simulink model "Lab6dff"  (R2016b)
settings: Solver=FixedStepAuto  StartTime=0.0  StopTime=20  FixedStep=0.01  RelTol=1e-3  EnableMultiTasking=on
values from neighbouring files (symbols this model uses):
  A = [0 a12 0 0;0 a22 a23 0;0 0 0 a34;0 a42 a43 0]    [Lab6d.m]    (also in data.mat = [0 0 0 0 1 -6.81227956989 0 15.4730759462 0 -1.49574193548 0; data2.mat = [0 0 0 0 1 -6.81227956989 0 15.4730759462 0 -1.49574193548 0; data3.mat = [0 0 0 0 1 -6.81227956989 0 15.4730759462 0 -1.49574193548 0; data4.mat = [0 0 0 0 1 -6.81227956989 0 15.4730759462 0 -1.49574193548 0)
  ang_thresh = 10*pi/180    (= 0.174532925199)    [Lab6d.m]    (also in data.mat; data2.mat; data3.mat; data4.mat)
  B = [0;b2;0;b4]    [Lab6d.m]    (also in data.mat = [0 1.52258064516 0 -3.45831460894]; data2.mat = [0 1.52258064516 0 -3.45831460894]; data3.mat = [0 1.52258064516 0 -3.45831460894]; data4.mat = [0 1.52258064516 0 -3.45831460894])
  C = [1 0 0 0;0 0 1 0]    [Lab6d.m]    (also in data.mat = [1  0  0  0; 0  0  1  0]; data2.mat = [1  0  0  0; 0  0  1  0]; data3.mat = [1  0  0  0; 0  0  1  0]; data4.mat = [1  0  0  0; 0  0  1  0])
  c_lp = 0.016    [Lab6d.m]    (also in data.mat; data2.mat; data3.mat; data4.mat)
  K = lqr(A,B,Q,R)    [Lab6d.m]    (also in data.mat = [-20 -39.3881221212 -301.165512499 -28.5227586286]; data2.mat = [-20 -39.3881221212 -301.165512499 -28.5227586286]; data3.mat = [-20 -39.3881221212 -301.165512499 -28.5227586286]; data4.mat = [-20 -39.3881221212 -301.165512499 -28.5227586286])
  K_pump = 300    [Lab6d.m]    (also in data.mat; data2.mat; data3.mat; data4.mat)
  L = place(A',C',po)'    [Lab6d.m]    (also in data.mat = [16.1595183214  -2.37669395577; 254.97799534  -5.48182894616; data2.mat = [16.1595183214  -2.37669395577; 254.97799534  -5.48182894616; data3.mat = [16.1595183214  -2.37669395577; 254.97799534  -5.48182894616; data4.mat = [16.1595183214  -2.37669395577; 254.97799534  -5.48182894616)
  ref = [0; 0; 0; 0]    [Lab6d.m]    (also in data.mat = [0 0 0 0]; data2.mat = [0 0 0 0]; data3.mat = [0.3 0 0 0]; data4.mat = [0.3 0 0 0])
  SAT = 4    [Lab6d.m]    (also in data.mat; data2.mat; data3.mat; data4.mat)
undefined symbols (not defined in the file or in its folder): HIL
libraries: quarc_library x3
settings Model: SimulationMode=external  Creator=ee128-aac  LastModifiedBy=ee105-abq
settings SolverCC: PositivePriorityOrder=on
settings RTWCC: SystemTargetFile=quarc_win64.tlc  TemplateMakefile=quarc_default_tmf  Description=QUARC Win64 Target
settings STFCustomTargetCC: TargetPreCompLibLocation=C:\PROGRA~3\QUARC\lib\2016b\win64\release  TargetLangStandard=C99 (ISO)  ConcurrentExecutionCompliant=on  SystemTargetFile=quarc_win64.tlc
settings GRTTargetCC: TargetPreCompLibLocation=C:\PROGRA~3\QUARC\lib\2016b\win64\release  ParMdlRefBuildCompliant=off  CompOptLevelCompliant=off  CombineOutputUpdateFcns=off  MatFileLogging=off  CPPClassGenCompliant=off  GRTInterface=on  UseToolchainInfoCompliant=off  ExtMode=on  ExtModeMexFile=quarc_comm

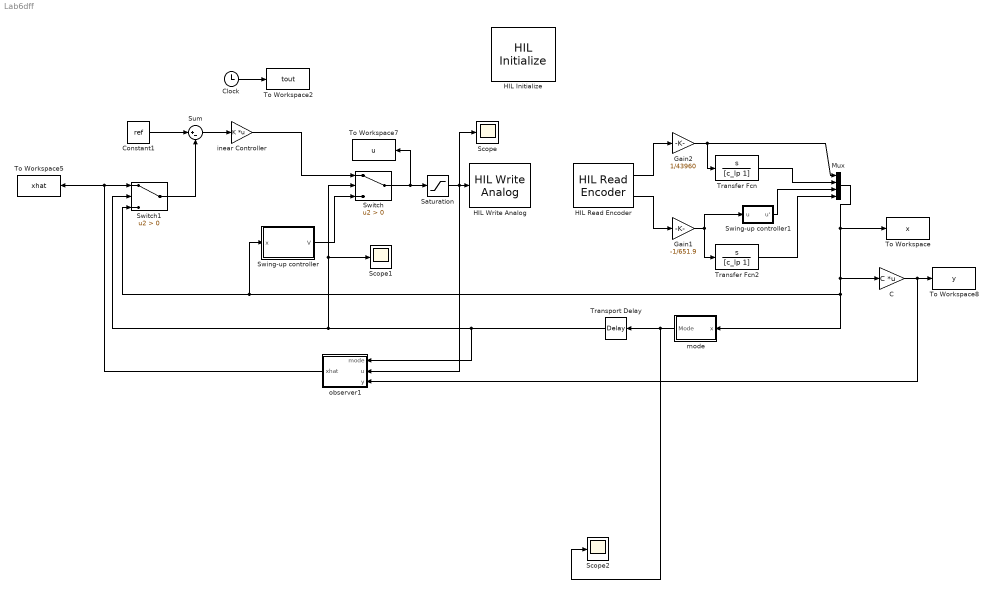
== system Lab6dff ==
  "C " : Gain  Gain=C  Multiplication=Matrix(K*u)
  Clock : Clock
  Constant1 : Constant  Value=ref
  Gain1 : Gain  Gain=-1/651.9
  Gain2 : Gain  Gain=1/43960
  HIL Initialize : quarc_library/Data Acquisition/Generic/Configuration/HIL Initialize  object_name=HIL-1  board_type=q4  board_number=0  board_options=""  exclusive=off  active=on  hardware_clocks=[0:1]  clock_modes=[0 0]  initial_clock_frequencies=[]  set_clock_params_at_start=on  set_clock_params_at_switch_in=off  set_clock_frequencies_at_start=off  set_clock_frequencies_at_switch_in=off  analog_input_channels=[0:3]  analog_input_configurations=[]  analog_input_maximums=10  analog_input_minimums=-10  set_analog_input_params_at_start=off  set_analog_input_params_at_switch_in=off  analog_output_channels=[0:3]  analog_output_maximums=[10]  analog_output_minimums=[-10]  initial_analog_outputs=[0]  final_analog_outputs=[0]  watchdog_analog_outputs=0  set_analog_output_params_at_start=on  set_analog_output_params_at_switch_in=off  set_analog_outputs_at_start=on  set_analog_outputs_at_switch_in=off  set_analog_outputs_at_terminate=on  set_analog_outputs_at_switch_out=off  set_analog_outputs_on_watchdog=off  digital_input_channels=[]  digital_output_channels=[]  digital_output_configuration=[]  initial_digital_outputs=[1]  final_digital_outputs=[1]  watchdog_digital_outputs=[2]  set_digital_output_params_at_start=off  set_digital_output_params_at_switch_in=off  set_digital_outputs_at_start=on  set_digital_outputs_at_switch_in=off  set_digital_outputs_at_terminate=on  set_digital_outputs_at_switch_out=off  set_digital_outputs_on_watchdog=off  encoder_channels=[0:3]  quadrature=[4]  encoder_filter_frequency=(1/60e-9)/1  initial_encoder_counts=[0]  set_encoder_params_at_start=on  set_encoder_params_at_switch_in=off  set_encoder_counts_at_start=on  set_encoder_counts_at_switch_in=off  pwm_channels=[]  pwm_modes=[0]  pwm_frequency=(1/60e-9)/1024  pwm_configuration=[]  pwm_alignment=[]  pwm_polarity=[]  pwm_leading_deadband=[]  pwm_trailing_deadband=[]  initial_pwm_outputs=[0]  final_pwm_outputs=[0]  watchdog_pwm_outputs=[]  set_pwm_params_at_start=on  set_pwm_params_at_switch_in=off  set_pwm_outputs_at_start=on  set_pwm_outputs_at_switch_in=off  set_pwm_outputs_at_terminate=on  set_pwm_outputs_at_switch_out=off  set_pwm_outputs_on_watchdog=off  other_output_channels=[]  initial_other_outputs=[]  final_other_outputs=[]  watchdog_other_outputs=[]  set_other_outputs_at_start=off  set_other_outputs_at_switch_in=off  set_other_outputs_at_terminate=off  set_other_outputs_at_switch_out=off  set_other_outputs_on_watchdog=off
  HIL Read Encoder : quarc_library/Data Acquisition/Generic/Immediate I//O/HIL Read Encoder  object_name=HIL-1  channels=[0:1]  sample_time=qc_get_step_size  active=on  vector_output=off  data_type_mode=Inherit via back propagation  data_type=double
  HIL Write Analog : quarc_library/Data Acquisition/Generic/Immediate I//O/HIL Write Analog  object_name=HIL-1  channels=[0]  sample_time=-1  active=off  vector_input=off
  Mux : Mux
  Saturation : Saturate  UpperLimit=6  LowerLimit=-6
  Scope : Scope
  Scope1 : Scope
  Scope2 : Scope
  Sum : Sum  Inputs=|+-
  Swing-up controller : Subsystem
  Swing-up controller1 : Subsystem
  Switch : Switch  Criteria=u2 > Threshold
  Switch1 : Switch  Criteria=u2 > Threshold
  To Workspace : ToWorkspace  VariableName=x  SampleTime=-1
  To Workspace2 : ToWorkspace  VariableName=tout  SampleTime=-1
  To Workspace5 : ToWorkspace  VariableName=xhat  SampleTime=-1
  To Workspace7 : ToWorkspace  VariableName=u  SampleTime=-1
  To Workspace8 : ToWorkspace  VariableName=y  SampleTime=-1
  Transfer Fcn : TransferFcn  Numerator=[1 0]  Denominator=[c_lp 1]
  Transfer Fcn2 : TransferFcn  Numerator=[1 0]  Denominator=[c_lp 1]
  Transport Delay : TransportDelay  DelayTime=0.25
  "inear Controller " : Gain  Gain=K  Multiplication=Matrix(K*u)
  mode : Subsystem
  observer1 : Subsystem
  wires:
  Saturation/1 -> observer1/2(u), HIL Write Analog/1, Scope/1
  HIL Read Encoder/1 -> Gain2/1
  HIL Read Encoder/2 -> Gain1/1
  Sum/1 -> "inear Controller "/1
  Gain1/1 -> Swing-up controller1/1(u), Transfer Fcn2/1
  Gain2/1 -> Transfer Fcn/1, Mux/1
  Clock/1 -> To Workspace2/1
  Mux/1 -> To Workspace/1, "C "/1, Switch1/3, Swing-up controller/1(x), mode/1(x)
  "C "/1 -> observer1/3(y), To Workspace8/1
  Transfer Fcn/1 -> Mux/2
  Transfer Fcn2/1 -> Mux/4
  mode/1(Mode) -> Scope2/1, Transport Delay/1
  Switch/1 -> To Workspace7/1, Saturation/1
  Swing-up controller/1(V) -> Switch/3
  "inear Controller "/1 -> Switch/1
  Constant1/1 -> Sum/1
  Switch1/1 -> Sum/2
  Transport Delay/1 -> observer1/1(mode), Scope1/1, Switch/2, Switch1/2
  observer1/1(xhat) -> To Workspace5/1, Switch1/1
  Swing-up controller1/1("u' ") -> Mux/3

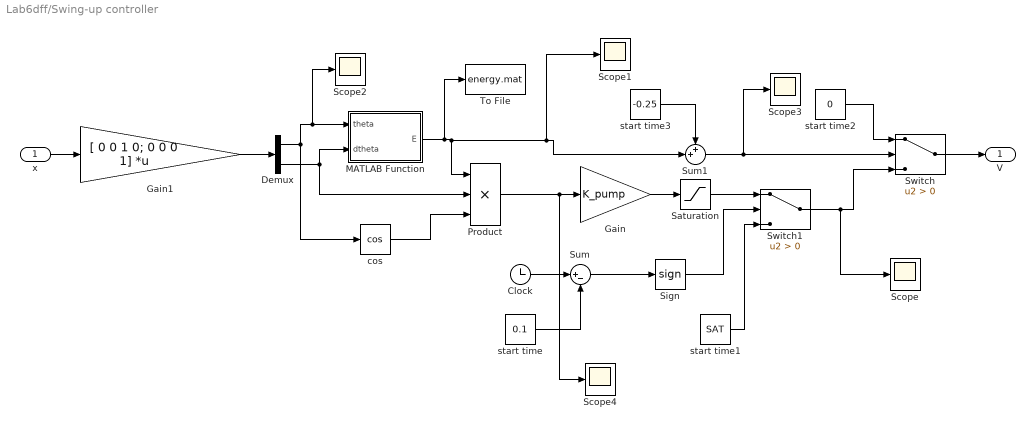
== system Lab6dff/Swing-up controller ==
  x : Inport
  Clock : Clock
      settings: Decimation=1000
  Demux : Demux  Outputs=2
  Gain : Gain  Gain=K_pump
  Gain1 : Gain  Gain=[ 0 0 1 0; 0 0 0 1]  Multiplication=Matrix(K*u)
  MATLAB Function : MATLAB Function  TreatAsAtomicUnit=on
  Product : Product  Inputs=3
  Saturation : Saturate  UpperLimit=6  LowerLimit=-6
  Scope{,1..4} (5 alike) : Scope
  Sign : Signum
  Sum : Sum  Inputs=|+-
  Sum1 : Sum  Inputs=++|
  Switch : Switch  Criteria=u2 > Threshold
  Switch1 : Switch  Criteria=u2 > Threshold
  To File : ToFile  Filename=energy.mat
  cos : Trigonometry  Operator=cos
  start time : Constant  Value=0.1
  start time1 : Constant  Value=SAT
  start time2 : Constant  Value=0
  start time3 : Constant  Value=-0.25
  V : Outport
  wires:
  Sum/1 -> Sign/1
  Clock/1 -> Sum/1
  start time/1 -> Sum/2
  Sign/1 -> Switch1/2
  start time1/1 -> Switch1/3
  Switch1/1 -> Scope/1, Switch/3
  Switch/1 -> V/1
  Saturation/1 -> Switch1/1
  Gain/1 -> Saturation/1
  Product/1 -> Scope4/1, Gain/1
  cos/1 -> Product/3
  x/1 -> Gain1/1
  Gain1/1 -> Demux/1
  Demux/2 -> MATLAB Function/2(dtheta), Product/2
  MATLAB Function/1(E) -> To File/1, Scope1/1, Sum1/2, Product/1
  start time2/1 -> Switch/1
  Demux/1 -> Scope2/1, MATLAB Function/1(theta), cos/1
  Sum1/1 -> Scope3/1, Switch/2
  start time3/1 -> Sum1/1

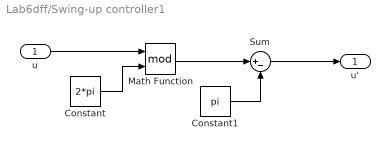
== system Lab6dff/Swing-up controller1 ==
  u : Inport
  Constant : Constant  Value=2*pi
  Constant1 : Constant  Value=pi
  Math Function : Math  Operator=mod  SaturateOnIntegerOverflow=on
  Sum : Sum  Inputs=|+-
  "u' " : Outport
  wires:
  u/1 -> Math Function/1
  Constant/1 -> Math Function/2
  Math Function/1 -> Sum/1
  Constant1/1 -> Sum/2
  Sum/1 -> "u' "/1

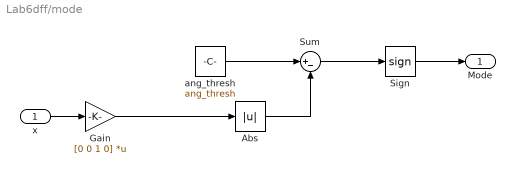
== system Lab6dff/mode ==
  x : Inport
  Abs : Abs
  Gain : Gain  Gain=[0 0 1 0]  Multiplication=Matrix(K*u)
  Sign : Signum
  Sum : Sum  Inputs=|+-
  ang_thresh : Constant  Value=ang_thresh
  Mode : Outport
  wires:
  Sign/1 -> Mode/1
  Sum/1 -> Sign/1
  Abs/1 -> Sum/2
  ang_thresh/1 -> Sum/1
  x/1 -> Gain/1
  Gain/1 -> Abs/1

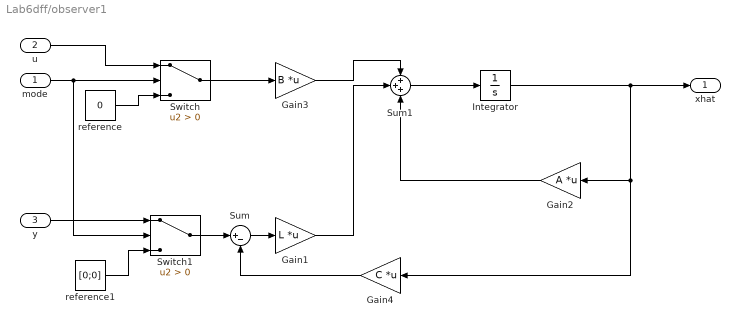
== system Lab6dff/observer1 ==
  mode : Inport
  u : Inport  Port=2
  y : Inport  Port=3
  Gain1 : Gain  Gain=L  Multiplication=Matrix(K*u)
  Gain2 : Gain  Gain=A  Multiplication=Matrix(K*u)
  Gain3 : Gain  Gain=B  Multiplication=Matrix(K*u)
  Gain4 : Gain  Gain=C  Multiplication=Matrix(K*u)
  Integrator : Integrator
  Sum : Sum  Inputs=|+-
  Sum1 : Sum  Inputs=+++
  Switch : Switch  Criteria=u2 > Threshold
  Switch1 : Switch  Criteria=u2 > Threshold
  reference : Constant  Value=0
  reference1 : Constant  Value=[0;0]
  xhat : Outport
  wires:
  u/1 -> Switch/1
  mode/1 -> Switch1/2, Switch/2
  reference/1 -> Switch/3
  y/1 -> Switch1/1
  reference1/1 -> Switch1/3
  Switch1/1 -> Sum/1
  Sum/1 -> Gain1/1
  Switch/1 -> Gain3/1
  Integrator/1 -> Gain4/1, Gain2/1, xhat/1
  Gain4/1 -> Sum/2
  Sum1/1 -> Integrator/1
  Gain3/1 -> Sum1/1
  Gain1/1 -> Sum1/2
  Gain2/1 -> Sum1/3

== matlab function Lab6dff/Swing-up controller/MATLAB Function ==
  data: theta input; E output; dtheta input
function E = fcn(theta,dtheta)
g=9.81;
m=0.23;
Lp=0.3302;
J = (4/3)*m*Lp^2;
E = 0.5*J*dtheta^2 + 1.9*m*g*Lp*(cos(theta)-1);
